simulink model "PM_fnc14a_DevHarness"  (R2022a)
settings: Solver=FixedStepDiscrete  StartTime=1  StopTime=inf  FixedStep=1  RelTol=1e-3
values from neighbouring files (symbols this model uses):
  fixedsteprate_s = rate_s    (= 0.01)    [PM_fnc1000_tc01_iter01_testsignal_builder.m]    (also in PM_fnc21_tc01_iter01_testsignal_builder.m; PM_fnc22_tc01_iter01_testsignal_builder.m)
undefined symbols (not defined in the file or in its folder): cal_DchgPL1_expiry_dur_thresh_ms, cal_DchgPL1_restore_dur_thresh_ms, cal_DchgPL2_expiry_dur_thresh_ms, cal_DchgPL2_restore_dur_thresh_ms, cal_table_cell_soc_percent, cal_table_cell_temp_degC, cal_table_DchgPL1_10s_limits_xtempysoc, cal_table_DchgPL1_60s_limits_xtempysoc, cal_table_DchgPL1_cont_limits_xtempysoc
libraries: PM_lib x3
settings Model: PacingRate=1.600000  Creator=306427  LastModifiedBy=306427
settings SolverCC: ZeroCrossAlgorithm=Adaptive

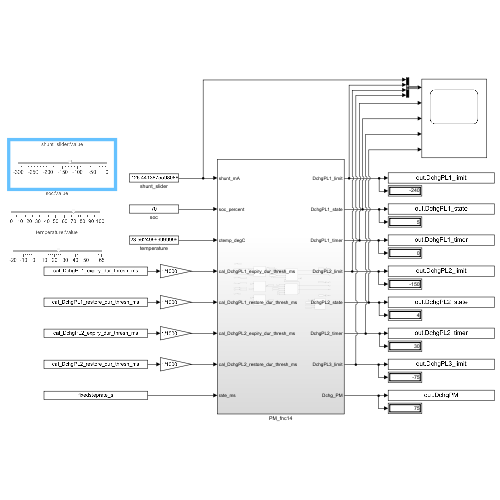
[thumbnail: Simulink's stored preview of the top-level diagram]
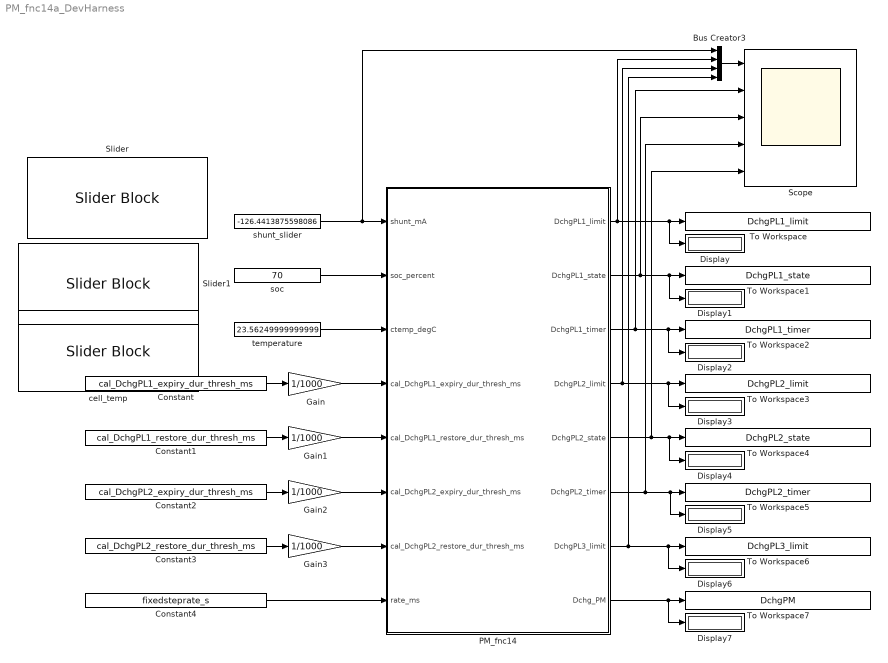
== system PM_fnc14a_DevHarness ==
  Bus Creator3 : BusCreator  Inputs=4
  Constant : Constant  Value=cal_DchgPL1_expiry_dur_thresh_ms
  Constant1 : Constant  Value=cal_DchgPL1_restore_dur_thresh_ms
  Constant2 : Constant  Value=cal_DchgPL2_expiry_dur_thresh_ms
  Constant3 : Constant  Value=cal_DchgPL2_restore_dur_thresh_ms
  Constant4 : Constant  Value=fixedsteprate_s
  Display{,1..7} (8 alike) : Display
  Gain{,1..3} (4 alike) : Gain  Gain=1/1000
  PM_fnc14 : Subsystem
  Scope : Scope  NumInputPorts=5
  Slider : SliderBlock  ScaleMin=-300  ScaleMax=0
  Slider1 : SliderBlock
  To Workspace : ToWorkspace  VariableName=DchgPL1_limit  SampleTime=-1
      settings: Save2DSignal=2-D array (concatenate along first dimension)
  To Workspace1 : ToWorkspace  VariableName=DchgPL1_state  SampleTime=-1
      settings: Save2DSignal=2-D array (concatenate along first dimension)
  To Workspace2 : ToWorkspace  VariableName=DchgPL1_timer  SampleTime=-1
      settings: Save2DSignal=2-D array (concatenate along first dimension)
  To Workspace3 : ToWorkspace  VariableName=DchgPL2_limit  SampleTime=-1
      settings: Save2DSignal=2-D array (concatenate along first dimension)
  To Workspace4 : ToWorkspace  VariableName=DchgPL2_state  SampleTime=-1
      settings: Save2DSignal=2-D array (concatenate along first dimension)
  To Workspace5 : ToWorkspace  VariableName=DchgPL2_timer  SampleTime=-1
      settings: Save2DSignal=2-D array (concatenate along first dimension)
  To Workspace6 : ToWorkspace  VariableName=DchgPL3_limit  SampleTime=-1
      settings: Save2DSignal=2-D array (concatenate along first dimension)
  To Workspace7 : ToWorkspace  VariableName=DchgPM  SampleTime=-1
      settings: Save2DSignal=2-D array (concatenate along first dimension)
  cell_temp : SliderBlock  ScaleMin=-20  ScaleMax=65
  shunt_slider : Constant  Value=-126.4413875598086
  soc : Constant  Value=70
  temperature : Constant  Value=23.56249999999999
  wires:
  soc/1 -> PM_fnc14/2(soc_percent)
  temperature/1 -> PM_fnc14/3(ctemp_degC)
  Constant/1 -> Gain/1
  Constant1/1 -> Gain1/1
  Constant2/1 -> Gain2/1
  Constant3/1 -> Gain3/1
  Constant4/1 -> PM_fnc14/8(rate_ms)
  shunt_slider/1 -> Bus Creator3/1, PM_fnc14/1(shunt_mA)
  PM_fnc14/1(DchgPL1_limit) -> Bus Creator3/2, Display/1, To Workspace/1
  PM_fnc14/2(DchgPL1_state) -> Display1/1, To Workspace1/1, Scope/3
  PM_fnc14/3(DchgPL1_timer) -> To Workspace2/1, Display2/1, Scope/2
  PM_fnc14/4(DchgPL2_limit) -> To Workspace3/1, Display3/1, Bus Creator3/3
  PM_fnc14/5(DchgPL2_state) -> Display4/1, To Workspace4/1, Scope/5
  PM_fnc14/7(DchgPL3_limit) -> Display6/1, To Workspace6/1, Bus Creator3/4
  Gain/1 -> PM_fnc14/4(cal_DchgPL1_expiry_dur_thresh_ms)
  Gain1/1 -> PM_fnc14/5(cal_DchgPL1_restore_dur_thresh_ms)
  Gain2/1 -> PM_fnc14/6(cal_DchgPL2_expiry_dur_thresh_ms)
  Gain3/1 -> PM_fnc14/7(cal_DchgPL2_restore_dur_thresh_ms)
  Bus Creator3/1 -> Scope/1
  PM_fnc14/6(DchgPL2_timer) -> Display5/1, To Workspace5/1, Scope/4
  PM_fnc14/8(Dchg_PM) -> Display7/1, To Workspace7/1

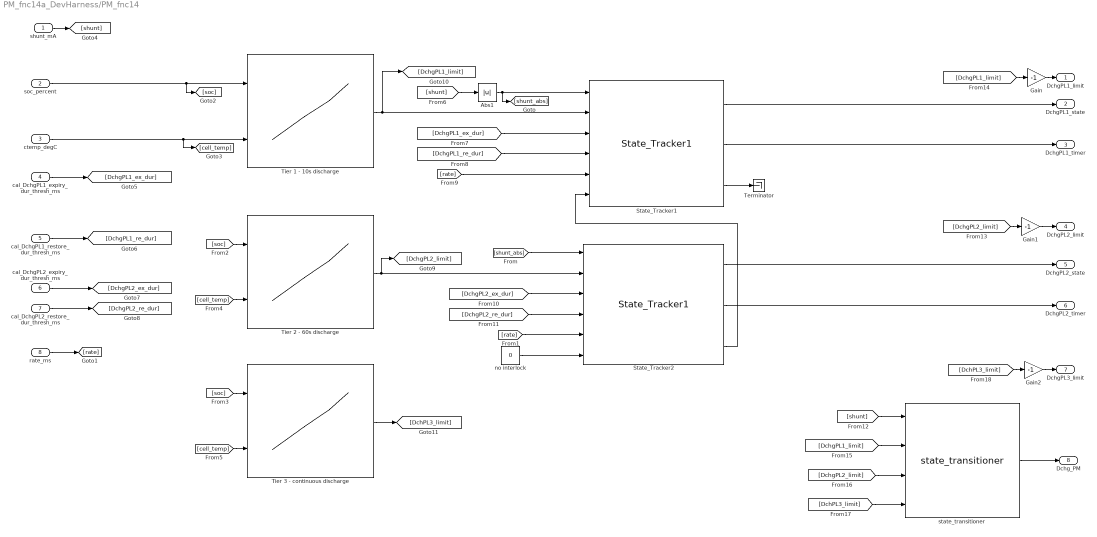
== system PM_fnc14a_DevHarness/PM_fnc14 ==
  shunt_mA : Inport
  soc_percent : Inport  Port=2
  ctemp_degC : Inport  Port=3
  cal_DchgPL1_expiry_dur_thresh_ms : Inport  Port=4
  cal_DchgPL1_restore_dur_thresh_ms : Inport  Port=5
  cal_DchgPL2_expiry_dur_thresh_ms : Inport  Port=6
  cal_DchgPL2_restore_dur_thresh_ms : Inport  Port=7
  rate_ms : Inport  Port=8
  Abs1 : Abs  SaturateOnIntegerOverflow=off
  Gain : Gain  Gain=-1
  Gain1 : Gain  Gain=-1
  Gain2 : Gain  Gain=-1
  State_Tracker1 : PM_lib/State_Tracker1  SystemSampleTime=-1  VariantActivationTime=update diagram  Latency=0  AutoFrameSizeCalculation=off
  State_Tracker2 : PM_lib/State_Tracker1  SystemSampleTime=-1  VariantActivationTime=update diagram  Latency=0  AutoFrameSizeCalculation=off
  Terminator : Terminator
  Tier 1 - 10s discharge : Lookup_n-D  BreakpointsForDimension1=cal_table_cell_soc_percent  BreakpointsForDimension2=cal_table_cell_temp_degC  Table=cal_table_DchgPL1_10s_limits_xtempysoc  InternalRulePriority=Speed  RndMeth=Simplest
      settings: InputPortMap=u0,u1
  Tier 2 - 60s discharge : Lookup_n-D  BreakpointsForDimension1=cal_table_cell_soc_percent  BreakpointsForDimension2=cal_table_cell_temp_degC  Table=cal_table_DchgPL1_60s_limits_xtempysoc  InternalRulePriority=Speed  RndMeth=Simplest
      settings: InputPortMap=u0,u1
  Tier 3 - continuous discharge : Lookup_n-D  BreakpointsForDimension1=cal_table_cell_soc_percent  BreakpointsForDimension2=cal_table_cell_temp_degC  Table=cal_table_DchgPL1_cont_limits_xtempysoc  InternalRulePriority=Speed  RndMeth=Simplest
      settings: InputPortMap=u0,u1
  no interlock : Constant  Value=0  OutDataTypeStr=boolean
  state_transitioner : PM_lib/state_transitioner  SystemSampleTime=-1  VariantActivationTime=update diagram  Latency=0  AutoFrameSizeCalculation=off
  DchgPL1_limit : Outport
  DchgPL1_state : Outport  Port=2
  DchgPL1_timer : Outport  Port=3
  DchgPL2_limit : Outport  Port=4
  DchgPL2_state : Outport  Port=5
  DchgPL2_timer : Outport  Port=6
  DchgPL3_limit : Outport  Port=7
  Dchg_PM : Outport  Port=8
  wires:
  [cell_temp] -> Tier 3 - continuous discharge/2
  State_Tracker2/2 -> DchgPL2_timer/1
  [soc] -> Tier 2 - 60s discharge/1
  [cell_temp] -> Tier 2 - 60s discharge/2
  ctemp_degC/1 -> [cell_temp], Tier 1 - 10s discharge/2
  [rate] -> State_Tracker1/5
  cal_DchgPL2_expiry_dur_thresh_ms/1 -> [DchgPL2_ex_dur]
  Tier 2 - 60s discharge/1 -> [DchgPL2_limit], State_Tracker2/2
  State_Tracker2/1 -> DchgPL2_state/1
  State_Tracker1/2 -> DchgPL1_timer/1
  State_Tracker1/1 -> DchgPL1_state/1
  [rate] -> State_Tracker2/5
  [soc] -> Tier 3 - continuous discharge/1
  rate_ms/1 -> [rate]
  cal_DchgPL1_expiry_dur_thresh_ms/1 -> [DchgPL1_ex_dur]
  [shunt_abs] -> State_Tracker2/1
  Abs1/1 -> State_Tracker1/1, [shunt_abs]
  shunt_mA/1 -> [shunt]
  cal_DchgPL1_restore_dur_thresh_ms/1 -> [DchgPL1_re_dur]
  Tier 1 - 10s discharge/1 -> [DchgPL1_limit], State_Tracker1/2
  soc_percent/1 -> [soc], Tier 1 - 10s discharge/1
  cal_DchgPL2_restore_dur_thresh_ms/1 -> [DchgPL2_re_dur]
  [shunt] -> Abs1/1
  [DchgPL2_re_dur] -> State_Tracker2/4
  [DchgPL2_ex_dur] -> State_Tracker2/3
  [DchgPL1_re_dur] -> State_Tracker1/4
  [DchgPL1_ex_dur] -> State_Tracker1/3
  no interlock/1 -> State_Tracker2/6
  State_Tracker2/3 -> State_Tracker1/6
  State_Tracker1/3 -> Terminator/1
  [shunt] -> state_transitioner/1
  state_transitioner/1 -> Dchg_PM/1
  [DchgPL2_limit] -> Gain1/1
  [DchgPL1_limit] -> Gain/1
  [DchgPL1_limit] -> state_transitioner/2
  [DchgPL2_limit] -> state_transitioner/3
  Tier 3 - continuous discharge/1 -> [DchPL3_limit]
  [DchPL3_limit] -> state_transitioner/4
  [DchPL3_limit] -> Gain2/1
  Gain/1 -> DchgPL1_limit/1
  Gain1/1 -> DchgPL2_limit/1
  Gain2/1 -> DchgPL3_limit/1
